simulink model "HANcoder_E407_SMV_program"  (R2018a)
settings: Solver=FixedStepDiscrete  StartTime=0.0  StopTime=1  FixedStep=0.01  RelTol=1e-3
PreLoadFcn:
  | librarySetup
  | eval([bdroot,'_startup']) %Calling [modelName]_startup.m
values from neighbouring files (symbols this model uses):
  Speed = [0.4; 0.4; 0.4; 0.4; 0.4; 0.4; 0.4; 0.4; 0.4; 0.4;0]    [Xbee_Track_Presentation.m]
undefined symbols (not defined in the file or in its folder): A0, A1, A2, A3, b, CON2, CON3, CON4, D13, D4, D5, drivemode, L_D1, L_D2, manual_xbee_switch, Steering_angle, steermode
libraries: HANcoder_STM32_Target x38, simulink_extras x11, simulink x7
(part 1 of 3)
CloseFcn:
  | rtwprivate ssgencode ModelCloseRequest mytest
settings Model: Creator=Jason van Kolfschoten  LastModifiedBy=abhik
settings SolverCC: PositivePriorityOrder=on
settings DataIOCC: LimitDataPoints=on  SaveFormat=Array  SignalLoggingSaveFormat=ModelDataLogs  SaveOutput=off  SaveTime=off
settings OptimizationCC: BlockReduction=off  DefaultParameterBehavior=Inlined  InlineInvariantSignals=on  ExpressionDepthLimit=2147483647  StateBitsets=on  DataBitsets=on  ZeroExternalMemoryAtStartup=off  ZeroInternalMemoryAtStartup=off  InitFltsAndDblsToZero=on  NoFixptDivByZeroProtection=on  EfficientFloat2IntCast=on  LifeSpan=inf
settings DebuggingCC: SaveWithDisabledLinksMsg=none  SaveWithParameterizedLinksMsg=none  CheckSSInitialOutputMsg=off  UnderspecifiedInitializationDetection=Classic  MergeDetectMultiDrivingBlocksExec=none  SignalResolutionControl=TryResolveAll  SolverPrmCheckMsg=warning  InheritedTsInSrcMsg=none  MultiTaskDSMMsg=warning  MultiTaskCondExecSysMsg=none  ParameterPrecisionLossMsg=none  FcnCallInpInsideContextMsg=warning  StateNameClashWarn=warning  SFUnexpectedBacktrackingDiag=warning  SFNoUnconditionalDefaultTransitionDiag=warning  SFExecutionAtInitializationDiag=none
settings HardwareCC: ProdBitPerPointer=32  ProdBitPerSizeT=32  ProdBitPerPtrDiffT=32  ProdLargestAtomicFloat=None  ProdIntDivRoundTo=Undefined  ProdWordSize=32  ProdHWDeviceType=Generic->32-bit Embedded Processor  TargetEndianess=LittleEndian  TargetHWDeviceType=Infineon->TriCore
settings ModelReferenceCC: PropagateSignalLabelsOutOfModel=off
settings SFSimCC: MATLABDynamicMemAlloc=off
settings RTWCC: SystemTargetFile=ert.tlc  MakeCommand=make_rtw SHELL= HANcoder_PORTABLE=1 HANcoder_BOOTLOADER=1  TemplateMakefile=STM32_E407_gcc.tmf  Description=Real-Time Workshop Embedded Coder (no auto configuration)
settings CodeAppCC: ForceParamTrailComments=on  IgnoreCustomStorageClasses=off  SimulinkDataObjDesc=on  CustomSymbolStrGlobalVar=rt$N$M  CustomSymbolStrType=$N$M  CustomSymbolStrFcn=$N$M$F  CustomSymbolStrMacro=$N$M  InsertBlockDesc=on  StateflowObjectComments=on  InternalIdentifier=Classic
settings ERTTargetCC: TargetFcnLib=ansi_tfl_tmw.mat  MultiwordLength=2048  IncludeMdlTerminateFcn=off  SuppressErrorStatus=on  SupportNonFinite=off  GenerateASAP2=on  InlinedParameterPlacement=NonHierarchical  ERTCustomFileTemplate=example_file_process.tlc  ConvertIfToSwitch=off  SuppressUnreachableDefaultCases=off
settings ConfigComp: CovMetricSettings=dw  CovHtmlReporting=on  CovSaveCumulativeToWorkspaceVar=on  CovSaveSingleToWorkspaceVar=on  CovExternalEMLEnable=off  DVMaxProcessTime=600  DVDisplayUnsatisfiableObjectives=on  DVAutomaticStubbing=off  DVModelCoverageObjectives=MCDC  DVMaxTestCaseSteps=500  DVTestSuiteOptimization=CombinedObjectives  DVDetectActiveLogic=on  DVDetectFloatOverflow=off  DVSaveHarnessModel=on

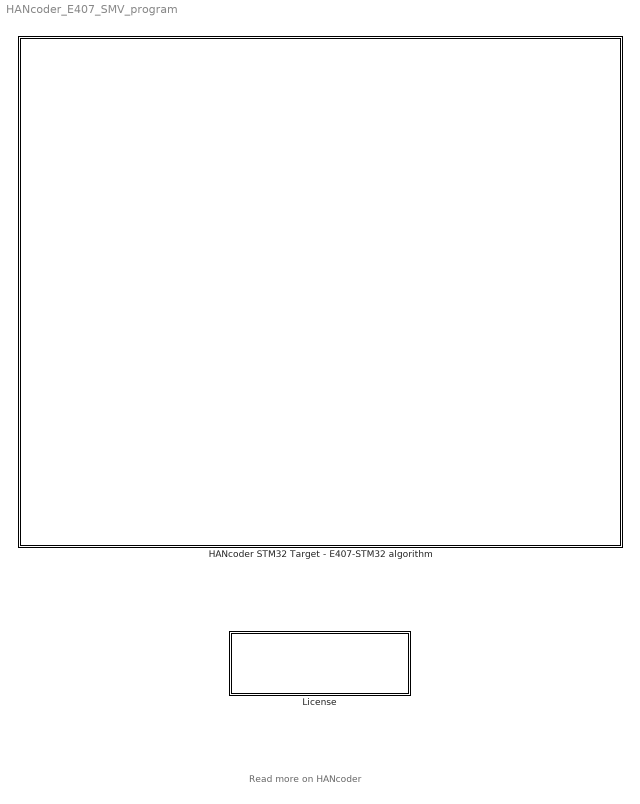
== system HANcoder_E407_SMV_program ==
  note: Read more on HANcoder
  HANcoder STM32 Target - E407-STM32 algorithm : Subsystem  mask(TopLevelSubsystem){}
      settings: CopyFcn=HANcoderChecks('Copy');  NameChangeFcn=HANcoderChecks('NameChangeE407');  MoveFcn=HANcoderChecks('MoveE407');
      mask Display: image(imread('STM32_E407_HAN.jpg'))
  License : Subsystem  mask(License){}
      settings: NameChangeFcn=HANcoderChecks('NameChangeLicenseBlock');  OpenFcn=winopen('License.pdf')  MoveFcn=HANcoderChecks('MoveLicenseBlock');
      mask Display: disp(['End-User License Agreement\n','please read before use']);

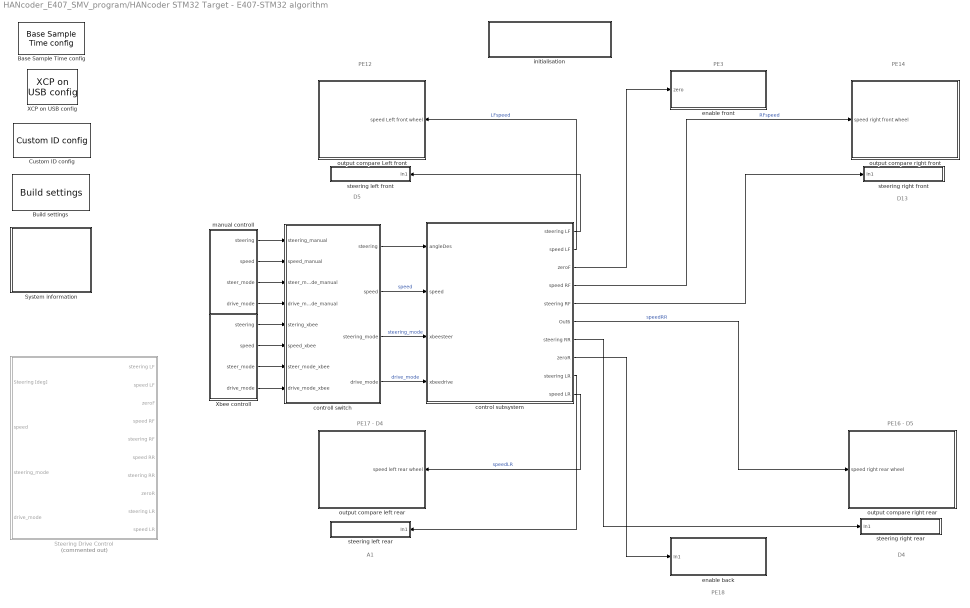
== system HANcoder_E407_SMV_program/HANcoder STM32 Target - E407-STM32 algorithm ==
  note: D4
  note: A1
  note: PE18
  note: PE3
  note: D13
  note: D5
  note: PE14
  note: PE16 - D5
  note: PE17 - D4
  note: PE12
  Base Sample Time config : HANcoder_STM32_Target/STM32-E407/System Config/Base Sample Time config  Tag=HANcoder_TARGET_STM32_E407  Description=HANcoder Target STM32-E407 blockset version 0.5  baseSampleTime=10  extraStack=0
      settings: SourceProductName=HANcoder STM32 Target
  Build settings : HANcoder_STM32_Target/STM32-E407/System Config/Build settings  Tag=HANcoder_TARGET_STM32_E407  AutoASAP2add=on  AutoFlash=USB
      settings: SourceProductName=HANcoder STM32 Target
  Custom ID config : HANcoder_STM32_Target/STM32-E407/System Config/Custom ID config  Tag=HANcoder_TARGET_STM32_E407  softID=softwareID  softNUM=1
      settings: SourceProductName=HANcoder STM32 Target
  Steering Drive Control : Subsystem  Commented=on
  System information : Subsystem
  XCP on USB config : HANcoder_STM32_Target/STM32-E407/System Config/XCP on USB config  Tag=HANcoder_TARGET_STM32_E407
      settings: SourceProductName=HANcoder STM32 Target
  Xbee controll : Subsystem
  control subsystem : Subsystem
  "controll switch " : Subsystem
  enable back : Subsystem
  enable front : Subsystem
  initialisation : Subsystem
  manual controll : Subsystem
  output compare Left front : Subsystem
  output compare left rear : Subsystem
  output compare right front : Subsystem
  output compare right rear : Subsystem
  steering left front : Subsystem
  steering left rear : Subsystem
  steering right front : Subsystem
  steering right rear : Subsystem
  wires:
  control subsystem/2(speed LF) -> output compare Left front/1(speed Left front wheel)  "LFspeed"
  control subsystem/4(speed RF) -> output compare right front/1(speed right front wheel)  "RFspeed"
  control subsystem/10(speed LR) -> output compare left rear/1(speed left rear wheel)  "speedLR"
  control subsystem/6(Out6) -> output compare right rear/1(speed right rear wheel)  "speedRR"
  control subsystem/3(zeroF) -> enable front/1(zero)
  control subsystem/8(zeroR) -> enable back/1(In1)
  control subsystem/5(steering RF) -> steering right front/1(In1)
  control subsystem/1(steering LF) -> steering left front/1(In1)
  control subsystem/7(steering RR) -> steering right rear/1(In1)
  control subsystem/9(steering LR) -> steering left rear/1(In1)
  "controll switch "/1(steering) -> control subsystem/1(angleDes)
  Xbee controll/3(steer_mode) -> "controll switch "/7(steer_mode_xbee)
  "controll switch "/2(speed) -> control subsystem/2(speed)  "speed"
  Xbee controll/1(steering) -> "controll switch "/5(stering_xbee)
  manual controll/4(drive_mode) -> "controll switch "/4(drive_mode_manual)
  "controll switch "/3(steering_mode) -> control subsystem/3(xbeesteer)  "steering_mode"
  manual controll/3(steer_mode) -> "controll switch "/3(steer_mode_manual)
  manual controll/2(speed) -> "controll switch "/2(speed_manual)
  Xbee controll/4(drive_mode) -> "controll switch "/8(drive_mode_xbee)
  "controll switch "/4(drive_mode) -> control subsystem/4(xbeedrive)  "drive_mode"
  Xbee controll/2(speed) -> "controll switch "/6(speed_xbee)
  manual controll/1(steering) -> "controll switch "/1(steering_manual)

== system HANcoder_E407_SMV_program/License ==

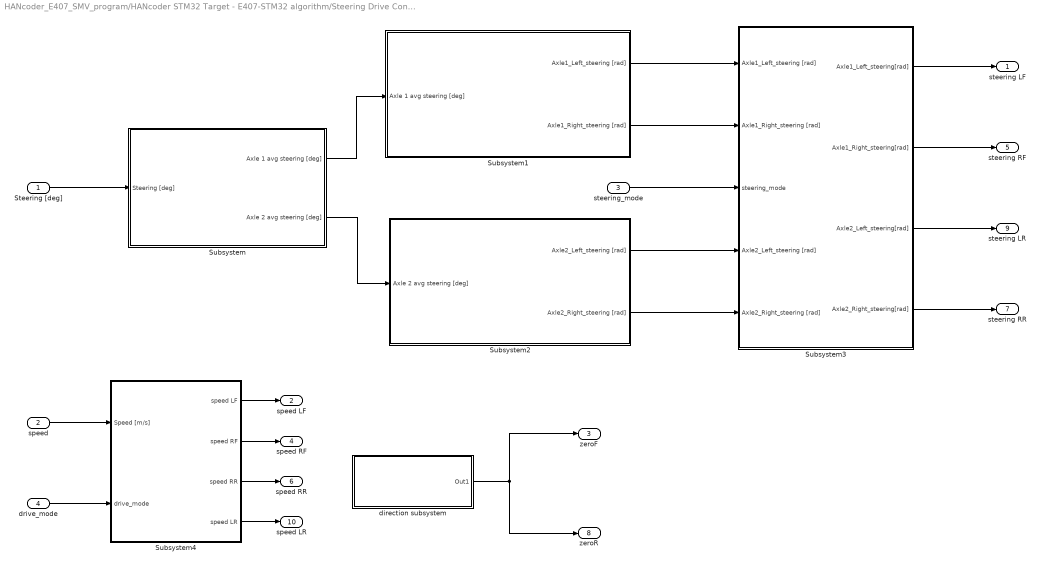
== system HANcoder_E407_SMV_program/HANcoder STM32 Target - E407-STM32 algorithm/Steering Drive Control ==
  Steering [deg] : Inport
  speed : Inport  Port=2
  steering_mode : Inport  Port=3
  drive_mode : Inport  Port=4
  Subsystem : Subsystem
  Subsystem1 : Subsystem
  Subsystem2 : Subsystem
  Subsystem3 : Subsystem
  Subsystem4 : Subsystem
  direction subsystem : Subsystem
  steering LF : Outport
  speed LF : Outport  Port=2
  zeroF : Outport  Port=3
  speed RF : Outport  Port=4
  steering RF : Outport  Port=5
  speed RR : Outport  Port=6
  steering RR : Outport  Port=7
  zeroR : Outport  Port=8
  steering LR : Outport  Port=9
  speed LR : Outport  Port=10
  wires:
  Steering [deg]/1 -> Subsystem/1(Steering [deg])
  Subsystem/1(Axle 1 avg steering [deg]) -> Subsystem1/1(Axle 1 avg steering [deg])
  Subsystem/2(Axle 2 avg steering [deg]) -> Subsystem2/1(Axle 2 avg steering [deg])
  steering_mode/1 -> Subsystem3/3(steering_mode)
  Subsystem1/1(Axle1_Left_steering [rad]) -> Subsystem3/1(Axle1_Left_steering [rad])
  Subsystem1/2(Axle1_Right_steering [rad]) -> Subsystem3/2(Axle1_Right_steering [rad])
  Subsystem2/1(Axle2_Left_steering [rad]) -> Subsystem3/4(Axle2_Left_steering [rad])
  Subsystem2/2(Axle2_Right_steering [rad]) -> Subsystem3/5(Axle2_Right_steering [rad])
  Subsystem3/1(Axle1_Left_steering[rad]) -> steering LF/1
  Subsystem3/2(Axle1_Right_steering[rad]) -> steering RF/1
  Subsystem3/3(Axle2_Left_steering[rad]) -> steering LR/1
  Subsystem3/4(Axle2_Right_steering[rad]) -> steering RR/1
  Subsystem4/1(speed LF) -> speed LF/1
  direction subsystem/1(Out1) -> zeroR/1, zeroF/1
  Subsystem4/2(speed RF) -> speed RF/1
  speed/1 -> Subsystem4/1(Speed [m/s])
  drive_mode/1 -> Subsystem4/2(drive_mode)
  Subsystem4/3(speed RR) -> speed RR/1
  Subsystem4/4(speed LR) -> speed LR/1

== system HANcoder_E407_SMV_program/HANcoder STM32 Target - E407-STM32 algorithm/System information ==
  note: These blocks check the free memory: stack and heap and the CPU load,
      | this way you can see whether your software demands too much of the microcontroller
  Get CPU load : HANcoder_STM32_Target/STM32-E407/System Management/Get CPU load  Tag=HANcoder_TARGET_STM32_E407  mode=Current CPU load  tsamp=-1
      settings: SourceProductName=HANcoder STM32 Target
  Get free Heap : HANcoder_STM32_Target/STM32-E407/System Management/Get free Heap  Tag=HANcoder_TARGET_STM32_E407  tsamp=-1
      settings: SourceProductName=HANcoder STM32 Target
  Get free Stack : HANcoder_STM32_Target/STM32-E407/System Management/Get free Stack  Tag=HANcoder_TARGET_STM32_E407  taskIdx=Application Control Task  tsamp=-1
      settings: SourceProductName=HANcoder STM32 Target
  Terminator : Terminator
  Terminator1 : Terminator
  Terminator2 : Terminator
  debug led : Subsystem
  wires:
  Get CPU load/1 -> Terminator1/1  "SI_CPUload"
  Get free Stack/1 -> Terminator/1  "SI_FreeStack"
  Get free Heap/1 -> Terminator2/1  "SI_FreeHeap"

== system HANcoder_E407_SMV_program/HANcoder STM32 Target - E407-STM32 algorithm/Xbee controll ==
  Check received data : Subsystem  TreatAsAtomicUnit=on
  Compare To Constant : simulink/Logic and Bit Operations/Compare To Constant  relop=>=  const=4  OutDataTypeStr=boolean
  Constant : Constant  Value=125
  Error value als het nodig is : Subsystem
  Gain : Gain  Gain=1/250
  Gain1 : Gain  Gain=1/4
  Rate Limiter1 : RateLimiter  RisingSlewLimit=0.25  FallingSlewLimit=-0.5  SampleTimeMode=inherited
  Rate Limiter2 : RateLimiter  RisingSlewLimit=100  FallingSlewLimit=-100  SampleTimeMode=inherited
  Sum : Sum  Inputs=|+-
  Switch : Switch  Criteria=u2 > Threshold
  UART receive buffer status : HANcoder_STM32_Target/STM32-E407/UART/UART receive buffer status  Tag=HANcoder_TARGET_STM32_E407  channel=UART1: CON3 - D1 & D0  tsamp=0.01
      settings: SourceProductName=HANcoder STM32 Target
  steering : Outport
  speed : Outport  Port=2
  steer_mode : Outport  Port=3
  drive_mode : Outport  Port=4
  wires:
  Check received data/2(Steering) -> Error value als het nodig is/2(SteeringIn)
  Compare To Constant/1 -> Check received data/Enable
  Check received data/1(Throttle) -> Error value als het nodig is/1(ThrottleIn)
  UART receive buffer status/1 -> Compare To Constant/1
  Error value als het nodig is/2(ThrottleOut) -> Gain/1
  Gain/1 -> Rate Limiter1/1
  Gain1/1 -> Rate Limiter2/1
  Sum/1 -> Gain1/1
  Constant/1 -> Sum/2, Switch/3
  Check received data/3(drive_mode) -> drive_mode/1
  Check received data/4(steer_mode) -> steer_mode/1
  Switch/1 -> Sum/1
  Error value als het nodig is/1(SteeringOut) -> Switch/2, Switch/1  "SteeringOut"
  Rate Limiter2/1 -> steering/1  "Steering"
  Rate Limiter1/1 -> speed/1

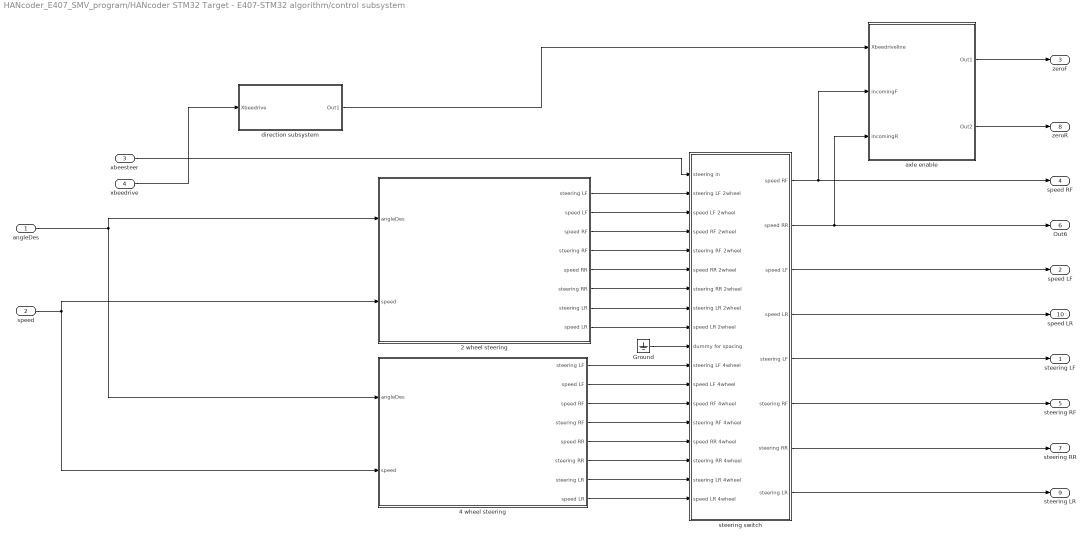
== system HANcoder_E407_SMV_program/HANcoder STM32 Target - E407-STM32 algorithm/control subsystem ==
  angleDes : Inport
  speed : Inport  Port=2
  xbeesteer : Inport  Port=3
  xbeedrive : Inport  Port=4
  2 wheel steering : Subsystem
  4 wheel steering : Subsystem
  Ground : Ground
  axle enable : Subsystem
  direction subsystem : Subsystem
  steering switch : Subsystem
  steering LF : Outport
  speed LF : Outport  Port=2
  zeroF : Outport  Port=3
  speed RF : Outport  Port=4
  steering RF : Outport  Port=5
  Out6 : Outport  Port=6
  steering RR : Outport  Port=7
  zeroR : Outport  Port=8
  steering LR : Outport  Port=9
  speed LR : Outport  Port=10
  wires:
  angleDes/1 -> 2 wheel steering/1(angleDes), 4 wheel steering/1(angleDes)
  xbeesteer/1 -> steering switch/1(steering in)
  2 wheel steering/1(steering LF) -> steering switch/2(steering LF 2wheel)
  2 wheel steering/2(speed LF) -> steering switch/3(speed LF 2wheel)
  2 wheel steering/3(speed RF) -> steering switch/4(speed RF 2wheel)
  2 wheel steering/4(steering RF) -> steering switch/5(steering RF 2wheel)
  2 wheel steering/5(speed RR) -> steering switch/6(speed RR 2wheel)
  2 wheel steering/6(steering RR) -> steering switch/7(steering RR 2wheel)
  2 wheel steering/7(steering LR) -> steering switch/8(steering LR 2wheel)
  2 wheel steering/8(speed LR) -> steering switch/9(speed LR 2wheel)
  4 wheel steering/1(steering LF) -> steering switch/11(steering LF 4wheel)
  4 wheel steering/2(speed LF) -> steering switch/12(speed LF 4wheel)
  4 wheel steering/3(speed RF) -> steering switch/13(speed RF 4wheel)
  4 wheel steering/4(steering RF) -> steering switch/14(steering RF 4wheel)
  4 wheel steering/5(speed RR) -> steering switch/15(speed RR 4wheel)
  4 wheel steering/6(steering RR) -> steering switch/16(steering RR 4wheel)
  4 wheel steering/7(steering LR) -> steering switch/17(steering LR 4wheel)
  4 wheel steering/8(speed LR) -> steering switch/18(speed LR 4wheel)
  steering switch/3(speed LF) -> speed LF/1
  steering switch/4(speed LR) -> speed LR/1
  steering switch/5(steering LF) -> steering LF/1
  steering switch/6(steering RF) -> steering RF/1
  steering switch/7(steering RR) -> steering RR/1
  steering switch/8(steering LR) -> steering LR/1
  Ground/1 -> steering switch/10(dummy for spacing)
  xbeedrive/1 -> direction subsystem/1(Xbeedrive)
  speed/1 -> 2 wheel steering/2(speed), 4 wheel steering/2(speed)
  steering switch/1(speed RF) -> axle enable/2(incomingF), speed RF/1
  steering switch/2(speed RR) -> axle enable/3(incomingR), Out6/1
  axle enable/1(Out1) -> zeroF/1
  axle enable/2(Out2) -> zeroR/1
  direction subsystem/1(Out1) -> axle enable/1(Xbeedriveline)

== system HANcoder_E407_SMV_program/HANcoder STM32 Target - E407-STM32 algorithm/controll switch  ==
  steering_manual : Inport
  speed_manual : Inport  Port=2
  steer_mode_manual : Inport  Port=3
  drive_mode_manual : Inport  Port=4
  stering_xbee : Inport  Port=5
  speed_xbee : Inport  Port=6
  steer_mode_xbee : Inport  Port=7
  drive_mode_xbee : Inport  Port=8
  3 = manual 1 = xbee : Constant  Value=manual_xbee_switch
  Switch{,1..3} (4 alike) : Switch  Criteria=u2 > Threshold  Threshold=2
  steering : Outport
  speed : Outport  Port=2
  steering_mode : Outport  Port=3
  drive_mode : Outport  Port=4
  wires:
  stering_xbee/1 -> Switch/3
  steering_manual/1 -> Switch/1
  speed_xbee/1 -> Switch1/3
  3 = manual 1 = xbee/1 -> Switch/2, Switch1/2, Switch3/2, Switch2/2
  Switch1/1 -> speed/1
  Switch/1 -> steering/1
  speed_manual/1 -> Switch1/1
  Switch3/1 -> drive_mode/1
  Switch2/1 -> steering_mode/1
  steer_mode_manual/1 -> Switch2/1
  drive_mode_manual/1 -> Switch3/1
  drive_mode_xbee/1 -> Switch3/3
  steer_mode_xbee/1 -> Switch2/3

== system HANcoder_E407_SMV_program/HANcoder STM32 Target - E407-STM32 algorithm/enable back ==
  In1 : Inport
  Digital Output : HANcoder_STM32_Target/STM32-E407/Digital Outputs/Digital Output  Tag=HANcoder_TARGET_STM32_E407  pinID=CON PE - 18  config=Push pull  tsamp=-1
      settings: SourceProductName=HANcoder STM32 Target
  wires:
  In1/1 -> Digital Output/1

== system HANcoder_E407_SMV_program/HANcoder STM32 Target - E407-STM32 algorithm/enable front ==
  zero : Inport
  Digital Output : HANcoder_STM32_Target/STM32-E407/Digital Outputs/Digital Output  Tag=HANcoder_TARGET_STM32_E407  pinID=CON PE - 3  config=Push pull  tsamp=-1
      settings: SourceProductName=HANcoder STM32 Target
  wires:
  zero/1 -> Digital Output/1

== system HANcoder_E407_SMV_program/HANcoder STM32 Target - E407-STM32 algorithm/initialisation ==
  note: 50 Hz ==> Period of 20 ms
      | Pusle width of 0.533 ms = 50 degrees
      | Pulse width of 2.235 ms = 180 degrees
  Output Compare Init1 : Subsystem  Tag=HANcoder_TARGET_STM32_E407  AncestorBlock=HANcoder_STM32_Target/STM32-E407/Timer Outputs/Output Compare Init  mask(Output Compare Init){moduleID=TIM1 - CON PE - 12 & 14 & 16 & 17, frequency=2000000, enableIRQoutput=off}
      mask prompts: moduleID "Timer module"; frequency "Frequency (free running counter) [Hz]"; enableIRQoutput "Enable IRQ output"
      mask help:
      | Function
      | ========
      | Initializes the timer module to allow output compare functionality on the
      | module's channels.
      |
      | Parameters
      | ==========
      | Timer Module:
      |   Selects the timer module.
      |
      | Frequency:
      |   Frequency at which the 16-bit free running counter counts.
      |
      | Enable IRQ output
      |   Controls whether or not the IRQ output is available.
      |
      | Outport
      | =======
      | IRQ
      |   Allows connection of a function call subsystem for the free running
      |   counter overflow event.
      mask init:
      | moduleIDInfoStr = sfcn_timeout_init_mcb(2, moduleID, frequency, enableIRQoutput);
      settings: CopyFcn=sfcn_timeout_init_chk();  MoveFcn=drawLogos
      mask Help: web('sfcn_timeout_init.html');
      mask TypeOptions moduleID: TIM1 - CON PE - 12 & 14 & 16 & 17 | TIM2 - CON4 - D13 & n/a & n/a & n/a | TIM3 - CON4 - D12 & D11 & n/a & n/a | TIM4 - CON PD - 15 & 16 &n/a & n/a | TIM8 - UEXT - 3 & 4 & n/a & n/a | TIM9 - CON3 - D4 & D5 or PE - 8 & 9 | TIM10 - CON2 - A1 or CON PF - 9 | TIM11 - CON2 - A2 or CON PF - 10 | TIM13 - CON2 - A3 or CON PF - 11 | TIM14 - CON2 - A4 or CON PF - 12
      mask Callback moduleID: sfcn_timeout_init_chk();
      mask Display: fprintf('Output Compare Init\n%s', moduleIDInfoStr);patch([195 201 201],[8 14 2],[1 0 0]);patch([203 203 209],[14 2 8],[0 0 0.35]);
  PWM Init : Subsystem  Tag=HANcoder_TARGET_STM32_E407  AncestorBlock=HANcoder_STM32_Target/STM32-E407/PWM Outputs/PWM Init  mask(Pulse Width Modulation Initialization){moduleID=TIM2:   D13 & n/a & n/a & n/a, frequency=50, alignment=Edge aligned, enableIRQoutput=off, ch1On=on, ch1Pol=Active high, ch1Inv=off, ch2On=on, ch2Pol=Active high, ch2Inv=off, ch3On=off, ch3Pol=Active high, ch3Inv=off, ch4On=off, ch4Pol=Active high, ch4Inv=off}
      mask prompts: moduleID "PWM module"; frequency "Signal frequency [Hz]"; alignment "Signal alignment"; enableIRQoutput "Enable IRQ output"; ch1On "Generate PWM signal on channel 1"; ch1Pol "Select signal polarity"; ch1Inv "Enable inverted signal on additional output pin"; ch2On "Generate PWM signal on channel 2"; ch2Pol "Select signal polarity"; ch2Inv "Enable inverted signal on additional output pin"; ch3On "Generate PWM signal on channel 3"; ch3Pol "Select signal polarity"; ch3Inv "Enable inverted signal on additional output pin"; ch4On "Generate PWM signal on channel 4"; ch4Pol "Select signal polarity"; ch4Inv "Enable inverted signal on additional output pin"
      mask help:
      | Function
      | ========
      | A 'PWM Init' block configures one of the STM32 timer modules for PWM
      | functionality, allowing a PWM signal to be generated on up to 4 timer
      | channels and their associated output pins.
      |
      | Parameters
      | ==========
      | General - PWM module:
      |   Select the PWM module to use. The name in the combo box contains
      |   information about which pins on the target belong to this timer module.
      |   Also the first pin corresponds with the first channel and so on:
      |   TIMx: Ch1 & Ch2 & Ch3...
      |
      | General - Signal frequency:
      |   Determines the signal frequency in Hz. If you click 'Apply' after entering
      |   the desired frequency it will automatically be adjusted to the closest
      |   supported value.
      |
      | General - Signal Aligment:
      |   Determines the aligment of the signal. It can either be edge aligned or
      |   center aligned.
      |
      | General - Enable IRQ output
      |   Controls whether or not the IRQ output is available.
      |
      | Channel x - Generate PWM signal on channel x:
      |   Enable to configure the channel for PWM functionality so that the PWM signal
      |   is outputted on the channel's associated microcontroller pin.
      |
      | Channel x - Signal polarity:
      |   Selects the polarity of the signal.
      |
      | Channel x - Enable inverted signal on additional output pin:
      |   When enabled, a second PWM signal will be generated on an additional
      |   microcontroller pin where the signal is an exact inversion of the first signal.
      mask init:
      | moduleIDInfoStr = sfcn_pwmout_init_mcb(2, moduleID, frequency, alignment, enableIRQoutput, ch1On, ch2On, ch3On, ch4On, ch1Pol, ch2Pol, ch3Pol, ch4Pol, ch1Inv, ch2Inv, ch3Inv, ch4Inv);
      settings: CopyFcn=sfcn_pwmout_init_chk();  MoveFcn=drawLogos
      mask Help: web('sfcn_pwmout_init.html');
      mask TypeOptions moduleID: TIM1:   PE12 & PE14 & PE16 & PE17 + N-channels PE11 & PE13 & PE15 | TIM2:   D13 & n/a & n/a & n/a | TIM3:   D12 & D11 & n/a & n/a | TIM4:   PD15 & PD16 &n/a & n/a | TIM8:   UEXT3 & UEXT4 & n/a & n/a | TIM9:   D4 & D5 & n/a & n/a | TIM10: A1 & n/a & n/a & n/a | TIM11: A2 & n/a & n/a & n/a | TIM13: A3 & n/a & n/a & n/a | TIM14: A4 & n/a & n/a & n/a
      mask Callback moduleID: sfcn_pwmout_init_chk();
      mask TypeOptions alignment: Edge aligned | Center aligned
      mask TypeOptions ch1Pol: Active high | Active low
      mask TypeOptions ch2Pol: Active high | Active low
      mask TypeOptions ch3Pol: Active high | Active low
      mask TypeOptions ch4Pol: Active high | Active low
      mask Display: fprintf('PWM Init\n%s', moduleIDInfoStr);patch([210 216 216],[8 14 2],[1 0 0]);patch([218 218 224],[14 2 8],[0 0 0.35]);
  PWM Init1 : Subsystem  Tag=HANcoder_TARGET_STM32_E407  AncestorBlock=HANcoder_STM32_Target/STM32-E407/PWM Outputs/PWM Init  mask(Pulse Width Modulation Initialization){moduleID=TIM9:   D4 & D5 & n/a & n/a, frequency=50, alignment=Edge aligned, enableIRQoutput=off, ch1On=on, ch1Pol=Active high, ch1Inv=off, ch2On=on, ch2Pol=Active high, ch2Inv=off, ch3On=off, ch3Pol=Active high, ch3Inv=off, ch4On=off, ch4Pol=Active high, ch4Inv=off}
      mask prompts: moduleID "PWM module"; frequency "Signal frequency [Hz]"; alignment "Signal alignment"; enableIRQoutput "Enable IRQ output"; ch1On "Generate PWM signal on channel 1"; ch1Pol "Select signal polarity"; ch1Inv "Enable inverted signal on additional output pin"; ch2On "Generate PWM signal on channel 2"; ch2Pol "Select signal polarity"; ch2Inv "Enable inverted signal on additional output pin"; ch3On "Generate PWM signal on channel 3"; ch3Pol "Select signal polarity"; ch3Inv "Enable inverted signal on additional output pin"; ch4On "Generate PWM signal on channel 4"; ch4Pol "Select signal polarity"; ch4Inv "Enable inverted signal on additional output pin"
      mask help:
      | Function
      | ========
      | A 'PWM Init' block configures one of the STM32 timer modules for PWM
      | functionality, allowing a PWM signal to be generated on up to 4 timer
      | channels and their associated output pins.
      |
      | Parameters
      | ==========
      | General - PWM module:
      |   Select the PWM module to use. The name in the combo box contains
      |   information about which pins on the target belong to this timer module.
      |   Also the first pin corresponds with the first channel and so on:
      |   TIMx: Ch1 & Ch2 & Ch3...
      |
      | General - Signal frequency:
      |   Determines the signal frequency in Hz. If you click 'Apply' after entering
      |   the desired frequency it will automatically be adjusted to the closest
      |   supported value.
      |
      | General - Signal Aligment:
      |   Determines the aligment of the signal. It can either be edge aligned or
      |   center aligned.
      |
      | General - Enable IRQ output
      |   Controls whether or not the IRQ output is available.
      |
      | Channel x - Generate PWM signal on channel x:
      |   Enable to configure the channel for PWM functionality so that the PWM signal
      |   is outputted on the channel's associated microcontroller pin.
      |
      | Channel x - Signal polarity:
      |   Selects the polarity of the signal.
      |
      | Channel x - Enable inverted signal on additional output pin:
      |   When enabled, a second PWM signal will be generated on an additional
      |   microcontroller pin where the signal is an exact inversion of the first signal.
      mask init:
      | moduleIDInfoStr = sfcn_pwmout_init_mcb(2, moduleID, frequency, alignment, enableIRQoutput, ch1On, ch2On, ch3On, ch4On, ch1Pol, ch2Pol, ch3Pol, ch4Pol, ch1Inv, ch2Inv, ch3Inv, ch4Inv);
      settings: CopyFcn=sfcn_pwmout_init_chk();  MoveFcn=drawLogos
      mask Help: web('sfcn_pwmout_init.html');
      mask TypeOptions moduleID: TIM1:   PE12 & PE14 & PE16 & PE17 + N-channels PE11 & PE13 & PE15 | TIM2:   D13 & n/a & n/a & n/a | TIM3:   D12 & D11 & n/a & n/a | TIM4:   PD15 & PD16 &n/a & n/a | TIM8:   UEXT3 & UEXT4 & n/a & n/a | TIM9:   D4 & D5 & n/a & n/a | TIM10: A1 & n/a & n/a & n/a | TIM11: A2 & n/a & n/a & n/a | TIM13: A3 & n/a & n/a & n/a | TIM14: A4 & n/a & n/a & n/a
      mask Callback moduleID: sfcn_pwmout_init_chk();
      mask TypeOptions alignment: Edge aligned | Center aligned
      mask TypeOptions ch1Pol: Active high | Active low
      mask TypeOptions ch2Pol: Active high | Active low
      mask TypeOptions ch3Pol: Active high | Active low
      mask TypeOptions ch4Pol: Active high | Active low
      mask Display: fprintf('PWM Init\n%s', moduleIDInfoStr);patch([210 216 216],[8 14 2],[1 0 0]);patch([218 218 224],[14 2 8],[0 0 0.35]);
  PWM Init2 : Subsystem  Tag=HANcoder_TARGET_STM32_E407  AncestorBlock=HANcoder_STM32_Target/STM32-E407/PWM Outputs/PWM Init  mask(Pulse Width Modulation Initialization){moduleID=TIM10: A1 & n/a & n/a & n/a, frequency=50, alignment=Edge aligned, enableIRQoutput=off, ch1On=on, ch1Pol=Active high, ch1Inv=off, ch2On=on, ch2Pol=Active high, ch2Inv=off, ch3On=off, ch3Pol=Active high, ch3Inv=off, ch4On=off, ch4Pol=Active high, ch4Inv=off}
      mask prompts: moduleID "PWM module"; frequency "Signal frequency [Hz]"; alignment "Signal alignment"; enableIRQoutput "Enable IRQ output"; ch1On "Generate PWM signal on channel 1"; ch1Pol "Select signal polarity"; ch1Inv "Enable inverted signal on additional output pin"; ch2On "Generate PWM signal on channel 2"; ch2Pol "Select signal polarity"; ch2Inv "Enable inverted signal on additional output pin"; ch3On "Generate PWM signal on channel 3"; ch3Pol "Select signal polarity"; ch3Inv "Enable inverted signal on additional output pin"; ch4On "Generate PWM signal on channel 4"; ch4Pol "Select signal polarity"; ch4Inv "Enable inverted signal on additional output pin"
      mask help:
      | Function
      | ========
      | A 'PWM Init' block configures one of the STM32 timer modules for PWM
      | functionality, allowing a PWM signal to be generated on up to 4 timer
      | channels and their associated output pins.
      |
      | Parameters
      | ==========
      | General - PWM module:
      |   Select the PWM module to use. The name in the combo box contains
      |   information about which pins on the target belong to this timer module.
      |   Also the first pin corresponds with the first channel and so on:
      |   TIMx: Ch1 & Ch2 & Ch3...
      |
      | General - Signal frequency:
      |   Determines the signal frequency in Hz. If you click 'Apply' after entering
      |   the desired frequency it will automatically be adjusted to the closest
      |   supported value.
      |
      | General - Signal Aligment:
      |   Determines the aligment of the signal. It can either be edge aligned or
      |   center aligned.
      |
      | General - Enable IRQ output
      |   Controls whether or not the IRQ output is available.
      |
      | Channel x - Generate PWM signal on channel x:
      |   Enable to configure the channel for PWM functionality so that the PWM signal
      |   is outputted on the channel's associated microcontroller pin.
      |
      | Channel x - Signal polarity:
      |   Selects the polarity of the signal.
      |
      | Channel x - Enable inverted signal on additional output pin:
      |   When enabled, a second PWM signal will be generated on an additional
      |   microcontroller pin where the signal is an exact inversion of the first signal.
      mask init:
      | moduleIDInfoStr = sfcn_pwmout_init_mcb(2, moduleID, frequency, alignment, enableIRQoutput, ch1On, ch2On, ch3On, ch4On, ch1Pol, ch2Pol, ch3Pol, ch4Pol, ch1Inv, ch2Inv, ch3Inv, ch4Inv);
      settings: CopyFcn=sfcn_pwmout_init_chk();  MoveFcn=drawLogos
      mask Help: web('sfcn_pwmout_init.html');
      mask TypeOptions moduleID: TIM1:   PE12 & PE14 & PE16 & PE17 + N-channels PE11 & PE13 & PE15 | TIM2:   D13 & n/a & n/a & n/a | TIM3:   D12 & D11 & n/a & n/a | TIM4:   PD15 & PD16 &n/a & n/a | TIM8:   UEXT3 & UEXT4 & n/a & n/a | TIM9:   D4 & D5 & n/a & n/a | TIM10: A1 & n/a & n/a & n/a | TIM11: A2 & n/a & n/a & n/a | TIM13: A3 & n/a & n/a & n/a | TIM14: A4 & n/a & n/a & n/a
      mask Callback moduleID: sfcn_pwmout_init_chk();
      mask TypeOptions alignment: Edge aligned | Center aligned
      mask TypeOptions ch1Pol: Active high | Active low
      mask TypeOptions ch2Pol: Active high | Active low
      mask TypeOptions ch3Pol: Active high | Active low
      mask TypeOptions ch4Pol: Active high | Active low
      mask Display: fprintf('PWM Init\n%s', moduleIDInfoStr);patch([210 216 216],[8 14 2],[1 0 0]);patch([218 218 224],[14 2 8],[0 0 0.35]);
  UART init : Subsystem  Tag=HANcoder_TARGET_STM32_E407  AncestorBlock=HANcoder_STM32_Target/STM32-E407/UART/UART init  mask(UART init){channel=UART1: CON3 - D1 & D0, baudrate=57600, databits=8, parity=none, stopbits=1, txbufsize=10, rxbufsize=12, useStatusOut=off}
      mask prompts: baudrate "Baudrate (bit/s)"; txbufsize "Transmit buffer size"; rxbufsize "Receive buffer size"; useStatusOut "Use status output"
      mask help:
      | Function
      | ==========
      | Initialized a UART channel.
      |
      | Parameters per channel
      | ======================
      | - Select channel (TX & RX)
      | - Select baudrate
      | - Select number of databits
      | - Select parity
      | - Select number of stopbits
      | - Configure the size of the transmit buffer
      | - Configure the size of the reception buffer
      | - Enable/disable the status output port
      mask init:
      | uartChannelInfoStr = sfcn_uart_init_mcb(2, channel, baudrate, databits, parity, stopbits, txbufsize, rxbufsize, useStatusOut);
      settings: CopyFcn=sfcn_uart_init_chk();  MoveFcn=drawLogos
      mask Help: web('sfcn_uart_init.html')
      mask TypeOptions channel: UART1: CON3 - D1 & D0 | UART2: CON PD - 8 & 9 | UART3: CON PD - 11 & 12 | UART6: UEXT - 3 & 4
      mask Callback channel: sfcn_uart_init_chk();
      mask TypeOptions baudrate: 300 | 600 | 1200 | 2400 | 4800 | 9600 | 19200 | 38400 | 57600 | 115200
      mask TypeOptions databits: 8 | 9
      mask TypeOptions parity: none | even | odd
      mask TypeOptions stopbits: 1 | 2
      mask Display: fprintf('UART init\n%s', uartChannelInfoStr);patch([236 242 242],[8 14 2],[1 0 0]);patch([244 244 250],[14 2 8],[0 0 0.35]);

== system HANcoder_E407_SMV_program/HANcoder STM32 Target - E407-STM32 algorithm/manual controll ==
  Rate Limiter : RateLimiter  RisingSlewLimit=0.5  FallingSlewLimit=-0.5  SampleTimeMode=inherited
  Rate Limiter4 : RateLimiter  RisingSlewLimit=100  FallingSlewLimit=-100  SampleTimeMode=inherited
  Speed : Constant  Value=Speed
  Steering angle : Constant  Value=Steering_angle
  speedvalue : Constant  Value=drivemode
  steeringvalue : Constant  Value=steermode
  steering : Outport
  speed : Outport  Port=2
  steer_mode : Outport  Port=3
  drive_mode : Outport  Port=4
  wires:
  Speed/1 -> Rate Limiter/1
  Steering angle/1 -> Rate Limiter4/1
  steeringvalue/1 -> steer_mode/1
  speedvalue/1 -> drive_mode/1
  Rate Limiter4/1 -> steering/1
  Rate Limiter/1 -> speed/1

== system HANcoder_E407_SMV_program/HANcoder STM32 Target - E407-STM32 algorithm/output compare Left front ==
  speed Left front wheel : Inport
  Compare Event IRQ1 : HANcoder_STM32_Target/STM32-E407/Timer Outputs/Compare Event IRQ  Tag=HANcoder_TARGET_STM32_E407  pin=TIM1 - CON PE - 12 - 5V Tolerant
      settings: SourceProductName=HANcoder STM32 Target
  Subsystem2 : Subsystem
  calculated frequency : Subsystem
  ms to tick conversion : Subsystem
  start : Constant
  start scheduling for output compare : Subsystem
  wires:
  Compare Event IRQ1/1 -> Subsystem2/Trigger
  speed Left front wheel/1 -> ms to tick conversion/1(m/s)
  ms to tick conversion/1(Out1) -> calculated frequency/1(ticks), Subsystem2/1(In1)
  start/1 -> start scheduling for output compare/Trigger

== system HANcoder_E407_SMV_program/HANcoder STM32 Target - E407-STM32 algorithm/output compare left rear ==
  speed left rear wheel : Inport
  Compare Event IRQ1 : HANcoder_STM32_Target/STM32-E407/Timer Outputs/Compare Event IRQ  Tag=HANcoder_TARGET_STM32_E407  pin=TIM1 - CON PE - 17 - 5V Tolerant
      settings: SourceProductName=HANcoder STM32 Target
  Subsystem2 : Subsystem
  Subsystem3 : Subsystem
  calculated frequency : Subsystem
  rad to tick conversion : Subsystem
  start : Constant
  wires:
  Compare Event IRQ1/1 -> Subsystem2/Trigger
  speed left rear wheel/1 -> rad to tick conversion/1(In1)
  start/1 -> Subsystem3/Trigger
  rad to tick conversion/1(Out1) -> calculated frequency/1(ticks), Subsystem2/1(In1)

== system HANcoder_E407_SMV_program/HANcoder STM32 Target - E407-STM32 algorithm/output compare right front ==
  speed right front wheel : Inport
  Compare Event IRQ1 : HANcoder_STM32_Target/STM32-E407/Timer Outputs/Compare Event IRQ  Tag=HANcoder_TARGET_STM32_E407  pin=TIM1 - CON PE - 14 - 5V Tolerant
      settings: SourceProductName=HANcoder STM32 Target
  Subsystem2 : Subsystem
  Subsystem3 : Subsystem
  calculated frequency : Subsystem
  rad to tick conversion : Subsystem
  start : Constant
  wires:
  Compare Event IRQ1/1 -> Subsystem2/Trigger
  rad to tick conversion/1(Out1) -> calculated frequency/1(ticks), Subsystem2/1(In1)
  speed right front wheel/1 -> rad to tick conversion/1(In1)
  start/1 -> Subsystem3/Trigger

== system HANcoder_E407_SMV_program/HANcoder STM32 Target - E407-STM32 algorithm/output compare right rear ==
  speed right rear wheel : Inport
  Compare Event IRQ1 : HANcoder_STM32_Target/STM32-E407/Timer Outputs/Compare Event IRQ  Tag=HANcoder_TARGET_STM32_E407  pin=TIM1 - CON PE - 16 - 5V Tolerant
      settings: SourceProductName=HANcoder STM32 Target
  Subsystem2 : Subsystem
  Subsystem3 : Subsystem
  calculated frequency : Subsystem
  ms to tick conversion : Subsystem
  start : Constant
  wires:
  Compare Event IRQ1/1 -> Subsystem2/Trigger
  start/1 -> Subsystem3/Trigger
  ms to tick conversion/1(Out1) -> calculated frequency/1(ticks), Subsystem2/1(In1)
  speed right rear wheel/1 -> ms to tick conversion/1(In1)

== system HANcoder_E407_SMV_program/HANcoder STM32 Target - E407-STM32 algorithm/steering left front ==
  note: Only true for angles between 50 and 180 degrees
  note: Only true for angles between 50 and 180 degrees
  In1 : Inport
  Add1 : Sum
  Analog Input : HANcoder_STM32_Target/STM32-E407/Analog Inputs/Analog Input  Tag=HANcoder_TARGET_STM32_E407  pinID=CON2 - A0  tsamp=-1  filtered=off
      settings: SourceProductName=HANcoder STM32 Target
  Constant : Constant  Value=108
  Constant1 : Constant  Value=101
  Data Type Conversion : DataTypeConversion  OutDataTypeStr=uint16
  Fcn : Fcn  Expr=0.67*u-6.16
  Gain : Gain  Gain=0.0586  OutDataTypeStr=uint16
  PWM Duty Cycle : HANcoder_STM32_Target/STM32-E407/PWM Outputs/PWM Duty Cycle  Tag=HANcoder_TARGET_STM32_E407  pinID=CON3 - D5  tsamp=-1
      settings: SourceProductName=HANcoder STM32 Target
  Sum1 : Sum  Inputs=|++
  Sum2 : Sum  Inputs=|+-
  Terminator : Terminator
  allignment tire : Constant  Value=-1
  wires:
  In1/1 -> Add1/2
  Data Type Conversion/1 -> PWM Duty Cycle/1
  Analog Input/1 -> Gain/1
  Fcn/1 -> Data Type Conversion/1
  Sum1/1 -> Fcn/1
  Constant/1 -> Sum1/2
  Constant1/1 -> Sum2/2
  Sum2/1 -> Terminator/1
  Gain/1 -> Sum2/1
  allignment tire/1 -> Add1/1
  Add1/1 -> Sum1/1

== system HANcoder_E407_SMV_program/HANcoder STM32 Target - E407-STM32 algorithm/steering left rear ==
  note: Only true for angles between 50 and 180 degrees
  note: Only true for angles between 50 and 180 degrees
  In1 : Inport
  Add3 : Sum
  Analog Input : HANcoder_STM32_Target/STM32-E407/Analog Inputs/Analog Input  Tag=HANcoder_TARGET_STM32_E407  pinID=CON2 - A2  tsamp=-1  filtered=off
      settings: SourceProductName=HANcoder STM32 Target
  Constant : Constant  Value=108
  Constant1 : Constant  Value=101
  Data Type Conversion : DataTypeConversion  OutDataTypeStr=uint16
  Fcn : Fcn  Expr=0.67*u-6.16
  Gain : Gain  Gain=0.0586  OutDataTypeStr=uint16
  PWM Duty Cycle : HANcoder_STM32_Target/STM32-E407/PWM Outputs/PWM Duty Cycle  Tag=HANcoder_TARGET_STM32_E407  pinID=CON2 - A1  tsamp=-1
      settings: SourceProductName=HANcoder STM32 Target
  Sum1 : Sum  Inputs=|++
  Sum2 : Sum  Inputs=|+-
  Terminator : Terminator
  allignment tire : Constant  Value=0
  wires:
  Analog Input/1 -> Gain/1
  Fcn/1 -> Data Type Conversion/1
  Data Type Conversion/1 -> PWM Duty Cycle/1
  Constant/1 -> Sum1/2
  Sum1/1 -> Fcn/1
  In1/1 -> Add3/2
  Constant1/1 -> Sum2/2
  Sum2/1 -> Terminator/1
  Gain/1 -> Sum2/1
  allignment tire/1 -> Add3/1
  Add3/1 -> Sum1/1

== system HANcoder_E407_SMV_program/HANcoder STM32 Target - E407-STM32 algorithm/steering right front ==
  note: Only true for angles between 50 and 180 degrees
  note: Only true for angles between 50 and 180 degrees
  In1 : Inport
  Add : Sum
  Analog Input : HANcoder_STM32_Target/STM32-E407/Analog Inputs/Analog Input  Tag=HANcoder_TARGET_STM32_E407  pinID=CON2 - A1  tsamp=-1  filtered=off
      settings: SourceProductName=HANcoder STM32 Target
  Constant : Constant  Value=108
  Constant1 : Constant  Value=101
  Data Type Conversion : DataTypeConversion  OutDataTypeStr=uint16
  Fcn : Fcn  Expr=0.67*u-6.16
  Gain : Gain  Gain=0.0586  OutDataTypeStr=uint16
  PWM Duty Cycle : HANcoder_STM32_Target/STM32-E407/PWM Outputs/PWM Duty Cycle  Tag=HANcoder_TARGET_STM32_E407  pinID=CON4 - D13  tsamp=-1
      settings: SourceProductName=HANcoder STM32 Target
  Sum1 : Sum  Inputs=|++
  Sum2 : Sum  Inputs=|+-
  Terminator : Terminator
  allignment tire : Constant
  wires:
  Data Type Conversion/1 -> PWM Duty Cycle/1
  Fcn/1 -> Data Type Conversion/1
  Analog Input/1 -> Gain/1
  Sum1/1 -> Fcn/1
  Constant/1 -> Sum1/2
  Constant1/1 -> Sum2/2
  Gain/1 -> Sum2/1
  Sum2/1 -> Terminator/1
  allignment tire/1 -> Add/1
  Add/1 -> Sum1/1
  In1/1 -> Add/2

== system HANcoder_E407_SMV_program/HANcoder STM32 Target - E407-STM32 algorithm/steering right rear ==
  note: Only true for angles between 50 and 180 degrees
  note: Only true for angles between 50 and 180 degrees
  In1 : Inport
  Add2 : Sum
  Analog Input : HANcoder_STM32_Target/STM32-E407/Analog Inputs/Analog Input  Tag=HANcoder_TARGET_STM32_E407  pinID=CON2 - A3  tsamp=-1  filtered=off
      settings: SourceProductName=HANcoder STM32 Target
  Constant : Constant  Value=108
  Constant1 : Constant  Value=101
  Data Type Conversion : DataTypeConversion  OutDataTypeStr=uint16
  Fcn : Fcn  Expr=0.67*u-6.16
  Gain : Gain  Gain=0.0586  OutDataTypeStr=uint16
  PWM Duty Cycle : HANcoder_STM32_Target/STM32-E407/PWM Outputs/PWM Duty Cycle  Tag=HANcoder_TARGET_STM32_E407  pinID=CON3 - D4  tsamp=-1
      settings: SourceProductName=HANcoder STM32 Target
  Sum1 : Sum  Inputs=|++
  Sum2 : Sum  Inputs=|+-
  Terminator : Terminator
  allignment tire : Constant  Value=2
  wires:
  Analog Input/1 -> Gain/1
  Fcn/1 -> Data Type Conversion/1
  Data Type Conversion/1 -> PWM Duty Cycle/1
  Constant/1 -> Sum1/2
  In1/1 -> Add2/2
  Sum1/1 -> Fcn/1
  Constant1/1 -> Sum2/2
  Gain/1 -> Sum2/1
  Sum2/1 -> Terminator/1
  allignment tire/1 -> Add2/1
  Add2/1 -> Sum1/1

== system HANcoder_E407_SMV_program/HANcoder STM32 Target - E407-STM32 algorithm/Steering Drive Control/Subsystem ==
  Steering [deg] : Inport
  Degrees to Radians : simulink_extras/Transformations/Degrees to Radians
  Distance of dolly first axle from pin coupling : Constant  Value=L_D1
  Distance of dolly second axle from pin coupling : Constant  Value=L_D2
  Divide : Product  Inputs=*/
  Divide1 : Product  Inputs=/*
  Fcn : Fcn  Expr=tan(u)
  Fcn1 : Fcn  Expr=atan(u)
  Fcn2 : Fcn  Expr=atan(u)
  Gain : Gain  Gain=1/2
  Multiply : Product
  Multiply1 : Product
  Sum : Sum
  Axle 1 avg steering [deg] : Outport
  Axle 2 avg steering [deg] : Outport  Port=2
  wires:
  Steering [deg]/1 -> Degrees to Radians/1
  Degrees to Radians/1 -> Fcn/1
  Distance of dolly first axle from pin coupling/1 -> Sum/1, Divide/1
  Distance of dolly second axle from pin coupling/1 -> Sum/2, Divide1/2
  Sum/1 -> Gain/1
  Gain/1 -> Divide/2, Divide1/1
  Divide/1 -> Multiply/2
  Divide1/1 -> Multiply1/1
  Fcn/1 -> Multiply1/2, Multiply/1
  Multiply/1 -> Fcn1/1
  Multiply1/1 -> Fcn2/1
  Fcn1/1 -> Axle 1 avg steering [deg]/1
  Fcn2/1 -> Axle 2 avg steering [deg]/1

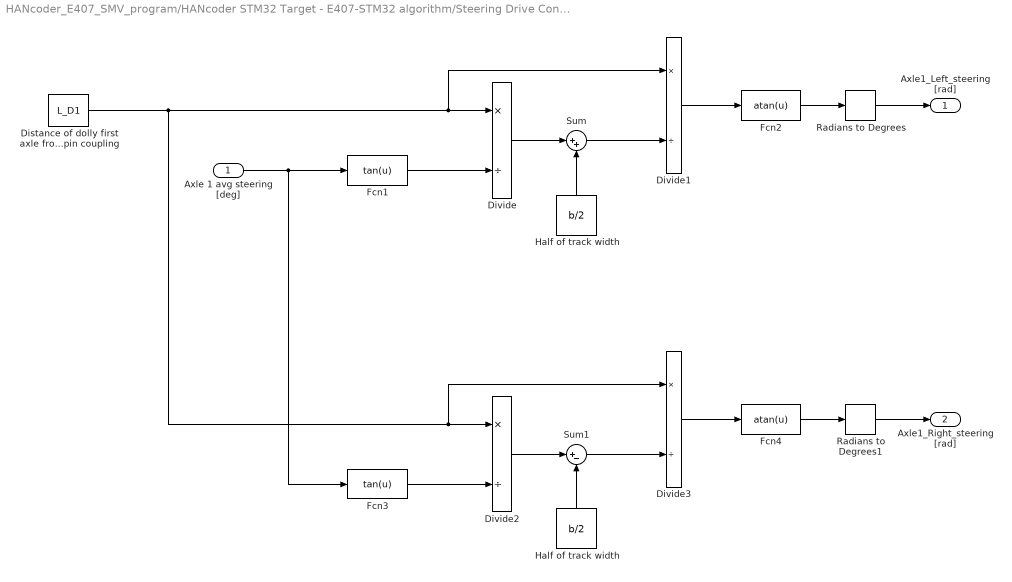
== system HANcoder_E407_SMV_program/HANcoder STM32 Target - E407-STM32 algorithm/Steering Drive Control/Subsystem1 ==
  Axle 1 avg steering [deg] : Inport
  Distance of dolly first axle from pin coupling : Constant  Value=L_D1
  Divide{,1..3} (4 alike) : Product  Inputs=*/
  Fcn1 : Fcn  Expr=tan(u)
  Fcn2 : Fcn  Expr=atan(u)
  Fcn3 : Fcn  Expr=tan(u)
  Fcn4 : Fcn  Expr=atan(u)
  Half of track width : Constant  Value=b/2  VectorParams1D=off  SampleTime=-1
  "Half of track width " : Constant  Value=b/2  VectorParams1D=off  SampleTime=-1
  Radians to Degrees : simulink_extras/Transformations/Radians to Degrees
  Radians to Degrees1 : simulink_extras/Transformations/Radians to Degrees
  Sum : Sum  Inputs=|++
  Sum1 : Sum  Inputs=|+-
  Axle1_Left_steering [rad] : Outport
  Axle1_Right_steering [rad] : Outport  Port=2
  wires:
  Fcn1/1 -> Divide/2
  Divide/1 -> Sum/1
  Sum/1 -> Divide1/2
  Half of track width/1 -> Sum/2
  Divide1/1 -> Fcn2/1
  Fcn2/1 -> Radians to Degrees/1
  Divide2/1 -> Sum1/1
  Fcn3/1 -> Divide2/2
  Distance of dolly first axle from pin coupling/1 -> Divide1/1, Divide/1, Divide3/1, Divide2/1
  Axle 1 avg steering [deg]/1 -> Fcn3/1, Fcn1/1
  Sum1/1 -> Divide3/2
  "Half of track width "/1 -> Sum1/2
  Divide3/1 -> Fcn4/1
  Fcn4/1 -> Radians to Degrees1/1
  Radians to Degrees/1 -> Axle1_Left_steering [rad]/1
  Radians to Degrees1/1 -> Axle1_Right_steering [rad]/1

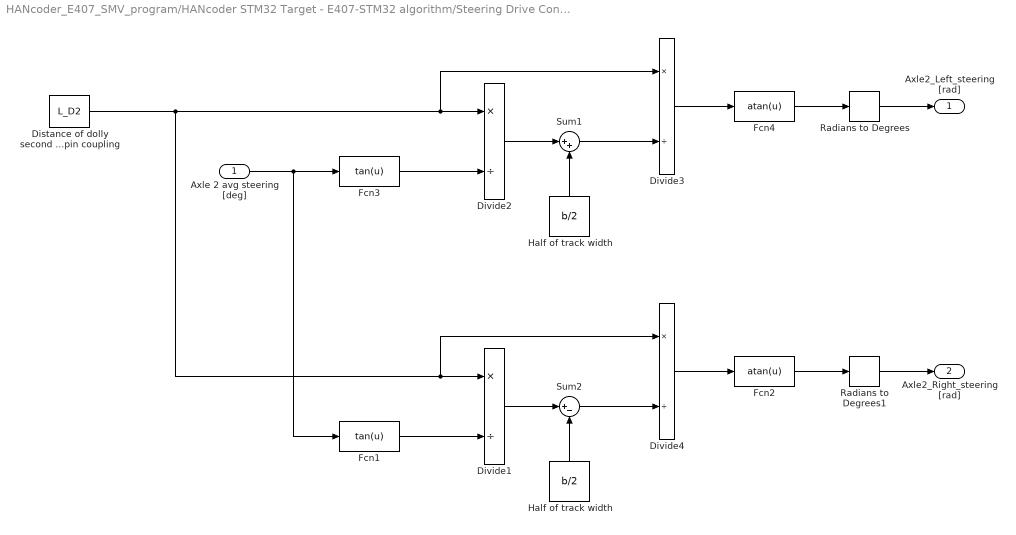
== system HANcoder_E407_SMV_program/HANcoder STM32 Target - E407-STM32 algorithm/Steering Drive Control/Subsystem2 ==
  Axle 2 avg steering [deg] : Inport
  Distance of dolly second axle from pin coupling : Constant  Value=L_D2
  Divide{1..4} (4 alike) : Product  Inputs=*/
  Fcn1 : Fcn  Expr=tan(u)
  Fcn2 : Fcn  Expr=atan(u)
  Fcn3 : Fcn  Expr=tan(u)
  Fcn4 : Fcn  Expr=atan(u)
  "Half of track width " : Constant  Value=b/2  VectorParams1D=off  SampleTime=-1
  "Half of track width  " : Constant  Value=b/2  VectorParams1D=off  SampleTime=-1
  Radians to Degrees : simulink_extras/Transformations/Radians to Degrees
  Radians to Degrees1 : simulink_extras/Transformations/Radians to Degrees
  Sum1 : Sum  Inputs=|++
  Sum2 : Sum  Inputs=|+-
  Axle2_Left_steering [rad] : Outport
  Axle2_Right_steering [rad] : Outport  Port=2
  wires:
  Fcn3/1 -> Divide2/2
  Divide2/1 -> Sum1/1
  Fcn4/1 -> Radians to Degrees/1
  Divide3/1 -> Fcn4/1
  "Half of track width "/1 -> Sum1/2
  Sum1/1 -> Divide3/2
  Sum2/1 -> Divide4/2
  "Half of track width  "/1 -> Sum2/2
  Divide4/1 -> Fcn2/1
  Fcn2/1 -> Radians to Degrees1/1
  Distance of dolly second axle from pin coupling/1 -> Divide4/1, Divide1/1, Divide2/1, Divide3/1
  Divide1/1 -> Sum2/1
  Fcn1/1 -> Divide1/2
  Axle 2 avg steering [deg]/1 -> Fcn1/1, Fcn3/1
  Radians to Degrees/1 -> Axle2_Left_steering [rad]/1
  Radians to Degrees1/1 -> Axle2_Right_steering [rad]/1

== system HANcoder_E407_SMV_program/HANcoder STM32 Target - E407-STM32 algorithm/Steering Drive Control/Subsystem3 ==
  Axle1_Left_steering [rad] : Inport
  Axle1_Right_steering [rad] : Inport  Port=2
  steering_mode : Inport  Port=3
  Axle2_Left_steering [rad] : Inport  Port=4
  Axle2_Right_steering [rad] : Inport  Port=5
  If : If  IfExpression=u1 == 1  ElseIfExpressions=u1 == 2, u1 == 3
  If Action Subsystem : Subsystem  TreatAsAtomicUnit=on
  If Action Subsystem1 : Subsystem  TreatAsAtomicUnit=on
  If Action Subsystem2 : Subsystem  TreatAsAtomicUnit=on
  If Action Subsystem3 : Subsystem  TreatAsAtomicUnit=on
  Merge{1..4} (4 alike) : Merge  Inputs=4
  Axle1_Left_steering[rad] : Outport
  Axle1_Right_steering[rad] : Outport  Port=2
  Axle2_Left_steering[rad] : Outport  Port=3
  Axle2_Right_steering[rad] : Outport  Port=4
  wires:
  steering_mode/1 -> If/1
  If/1 -> If Action Subsystem/Action
  If/2 -> If Action Subsystem1/Action
  If/3 -> If Action Subsystem2/Action
  Axle1_Left_steering [rad]/1 -> If Action Subsystem/1(Axle1_Left_steering [rad]), If Action Subsystem2/1(Axle1_Left_steering [rad])
  Axle2_Right_steering [rad]/1 -> If Action Subsystem1/2(Axle2_Right_steering [rad]), If Action Subsystem2/4(Axle2_Right_steering [rad])
  Axle2_Left_steering [rad]/1 -> If Action Subsystem1/1(Axle2_Left_steering [rad]), If Action Subsystem2/3(Axle2_Left_steering [rad])
  Axle1_Right_steering [rad]/1 -> If Action Subsystem/2(Axle1_Right_steering [rad]), If Action Subsystem2/2(Axle1_Right_steering [rad])
  If/4 -> If Action Subsystem3/Action
  If Action Subsystem3/4(Axle2_Right_steering[rad]) -> Merge3/4
  If Action Subsystem/4(Axle2_Right_steering[rad]) -> Merge3/1
  If Action Subsystem2/4(Axle2_Right_steering[rad]) -> Merge3/3
  If Action Subsystem1/4(Axle2_Right_steering[rad]) -> Merge3/2
  Merge3/1 -> Axle2_Right_steering[rad]/1
  If Action Subsystem3/3(Axle2_Left_steering[rad]) -> Merge1/4
  If Action Subsystem2/3(Axle2_Left_steering[rad]) -> Merge1/3
  If Action Subsystem1/3(Axle2_Left_steering[rad]) -> Merge1/2
  If Action Subsystem/3(Axle2_Left_steering[rad]) -> Merge1/1
  Merge1/1 -> Axle2_Left_steering[rad]/1
  If Action Subsystem3/2(Axle1_Right_steering[rad]) -> Merge2/4
  If Action Subsystem2/2(Axle1_Right_steering[rad]) -> Merge2/3
  If Action Subsystem1/2(Axle1_Right_steering[rad]) -> Merge2/2
  If Action Subsystem/2(Axle1_Right_steering[rad]) -> Merge2/1
  Merge2/1 -> Axle1_Right_steering[rad]/1
  If Action Subsystem3/1(Axle1_Left_steering[rad]) -> Merge4/4
  If Action Subsystem2/1(Axle1_Left_steering[rad]) -> Merge4/3
  If Action Subsystem1/1(Axle1_Left_steering[rad]) -> Merge4/2
  If Action Subsystem/1(Axle1_Left_steering[rad]) -> Merge4/1
  Merge4/1 -> Axle1_Left_steering[rad]/1

== system HANcoder_E407_SMV_program/HANcoder STM32 Target - E407-STM32 algorithm/Steering Drive Control/Subsystem4 ==
  Speed [m/s] : Inport
  drive_mode : Inport  Port=2
  If : If  IfExpression=u1 ==1  ShowElse=off
  If Action Subsystem : Subsystem  TreatAsAtomicUnit=on
  speed LF : Outport
  speed RF : Outport  Port=2
  speed RR : Outport  Port=3
  speed LR : Outport  Port=4
  wires:
  Speed [m/s]/1 -> If Action Subsystem/1(In1)
  If/1 -> If Action Subsystem/Action
  If Action Subsystem/1(Out1) -> speed LF/1, speed RF/1, speed RR/1, speed LR/1
  drive_mode/1 -> If/1

== system HANcoder_E407_SMV_program/HANcoder STM32 Target - E407-STM32 algorithm/Steering Drive Control/direction subsystem ==
  Constant : Constant  OutDataTypeStr=boolean
  Constant1 : Constant  OutDataTypeStr=boolean
  Digital Output1 : HANcoder_STM32_Target/STM32-E407/Digital Outputs/Digital Output  Tag=HANcoder_TARGET_STM32_E407  pinID=CON PE - 4  config=Push pull  tsamp=-1
      settings: SourceProductName=HANcoder STM32 Target
  Out1 : Outport
  wires:
  Constant/1 -> Digital Output1/1
  Constant1/1 -> Out1/1

== system HANcoder_E407_SMV_program/HANcoder STM32 Target - E407-STM32 algorithm/System information/debug led ==
  Algorithm : Subsystem
  Inputs : Subsystem
  Outputs : Subsystem
  wires:
  Inputs/1(Button) -> Algorithm/1(Button)
  Algorithm/1(LED) -> Outputs/1(LED)

== system HANcoder_E407_SMV_program/HANcoder STM32 Target - E407-STM32 algorithm/Xbee controll/Check received data ==
  note: Here we check if the start byte is the first byte in the buffer, if not it will read 1 byte and thus deleting this one from the buffer
  Enable : EnablePort
  Check next 3 bytes and send via CAN : Subsystem  TreatAsAtomicUnit=on
  Check received data : Subsystem  TreatAsAtomicUnit=on
  Switch Case : SwitchCase  CaseConditions={252,250}  ShowDefaultCase=off
  UART start : Subsystem  Tag=HANcoder_TARGET_STM32_E407  AncestorBlock=HANcoder_STM32_Target/STM32-E407/UART/UART receive  mask(UART receive){channel=UART1: CON3 - D1 & D0, useStatusOut=off, tsamp=-1}
      mask prompts: useStatusOut "Use status outport"; tsamp "Sample time"
      mask help:
      | Function
      | ==========
      | Reads a byte from the UART reception buffer.
      |
      | Parameters per channel
      | ======================
      | - Select channel (TX & RX)
      | - Select if the status output should be enabled.
      |
      | Outputs
      | =======
      | - The value of the receive byte.
      | - When the status output is 0, the reception buffer was empty.
      mask init:
      | uartChannelInfoStr = sfcn_uart_receive_mcb(2, channel, useStatusOut);
      settings: MoveFcn=drawLogos
      mask Help: web('sfcn_uart_receive.html')
      mask TypeOptions channel: UART1: CON3 - D1 & D0 | UART2: CON PD - 8 & 9 | UART3: CON PD - 11 & 12 | UART6: UEXT - 3 & 4
      mask Display: fprintf('UART receive\n%s', uartChannelInfoStr);patch([240 246 246],[8 14 2],[1 0 0]);patch([248 248 254],[14 2 8],[0 0 0.35]);
  Throttle : Outport
  Steering : Outport  Port=2
  drive_mode : Outport  Port=3
  steer_mode : Outport  Port=4
  wires:
  UART start/1(Out1) -> Switch Case/1
  Check next 3 bytes and send via CAN/1(Throttle) -> Throttle/1
  Switch Case/2 -> Check next 3 bytes and send via CAN/Action
  Switch Case/1 -> Check received data/Action
  Check received data/1(drive_mode) -> drive_mode/1
  Check received data/2(steer_mode) -> steer_mode/1
  Check next 3 bytes and send via CAN/2(Steering) -> Steering/1
